simulink model "testautosize"  (R2016a)
settings: Solver=VariableStepAuto  StartTime=0.0  StopTime=10.0  RelTol=1e-3
settings Model: Creator=eruffaldi  LastModifiedBy=eruffaldi

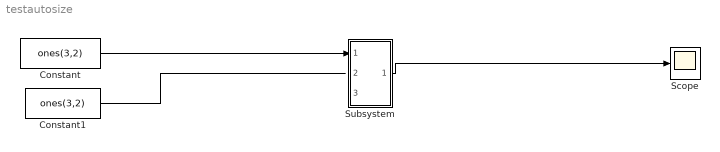
== system testautosize ==
  Constant : Constant  Value=ones(3,2)
  Constant1 : Constant  Value=ones(3,2)
  Scope : Scope
  Subsystem : Subsystem  mask{Inputs=3}
      mask Callback Inputs:
      | x = gcb;
      | s = gcb;
      | asked = max(1,str2num(get_param(gcb,'Inputs')));
      | 
      | bcon = [x '/Matrix Concatenate'];
      | actual = str2num(get_param(bcon,'NumInputs'));
      | 
      | if asked == actual
      | else
      | bconL = bcon(length(x)+2:end);
      | 
      | if asked > actual
      |     set_param(bcon,'NumInputs',num2str(asked));
      |     bin1 = ([x '/In1']);
      |     bsh1 = ([x '/Reshape1']);
      |     bin1L = bin1(length(x)+2:end);
      |     bsh1L = bsh1(length(x)+2:end);
      |     for I=actual+1:asked
      |         bin = sprintf([x '/In%d'],I);
      |         bsh = sprintf([x '/Reshape%d'],I);
      |         binL = bin(length(x)+2:end);
      |         bshL = bsh(length(x)+2:end);
      |         % clone In and Reshape
      |         add_block(bin1,bin);
      |         add_block(bsh1,bsh);
      |         add_line(s,[binL '/1'],[bshL '/1']);
      |         add_line(s,[bshL '/1'],[bconL sprintf('/%d',I)]);
      |     end
      | else
      |     % remove
      |     for I=actual:-1:asked+1
      |         bin = sprintf([x '/In%d'],I);
      |         bsh = sprintf([x '/Reshape%d'],I);
      |         binL = bin(length(x)+2:end);
      |         bshL = bsh(length(x)+2:end);
      | 
      |         try
      |         delete_line(s,[binL '/1'],[bshL '/1']);
      |         catch me
      |         end
      |         try
      |         delete_line(s,[bshL '/1'],[bconL sprintf('/%d',I)]);
      |         catch me
      |         end
      |         try
      |         delete_block(bin);
      |         catch me
      |         end
      |         try
      |         delete_block(bsh);
      |         catch me
      |         end
      |     end
      |     set_param(bcon,'NumInputs',num2str(asked));
      | end
      | end
  wires:
  Constant/1 -> Subsystem/1(In1)
  Subsystem/1(Out1) -> Scope/1
  Constant1/1 -> ?

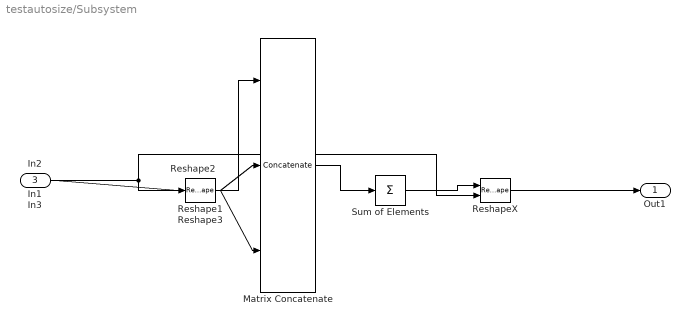
== system testautosize/Subsystem ==
  In1 : Inport
  In2 : Inport  Port=2
  In3 : Inport  Port=3
  Matrix Concatenate : Concatenate  NumInputs=3  Mode=Multidimensional array  ConcatenateDimension=2
  Reshape1 : Reshape
  Reshape2 : Reshape
  Reshape3 : Reshape
  ReshapeX : Reshape  OutputDimensionality=Derive from reference input port
  Sum of Elements : Sum  Inputs=+  CollapseMode=Specified dimension  CollapseDim=2
  Out1 : Outport
  wires:
  Sum of Elements/1 -> ReshapeX/1
  In1/1 -> ReshapeX/2, Reshape1/1
  Reshape1/1 -> Matrix Concatenate/1
  Matrix Concatenate/1 -> Sum of Elements/1
  ReshapeX/1 -> Out1/1
  In2/1 -> Reshape2/1
  Reshape2/1 -> Matrix Concatenate/2
  In3/1 -> Reshape3/1
  Reshape3/1 -> Matrix Concatenate/3
